simulink model "miniproject1901156"  (R2017b)
settings: Solver=VariableStepAuto  StartTime=0.0  StopTime=0.2  MaxStep=1e-4  RelTol=1e-3
undefined symbols (not defined in the file): D1, Delta
libraries: powerlib x32, powerlib_meascontrol x3
settings Model: Creator=DVCBD  LastModifiedBy=DVCBD

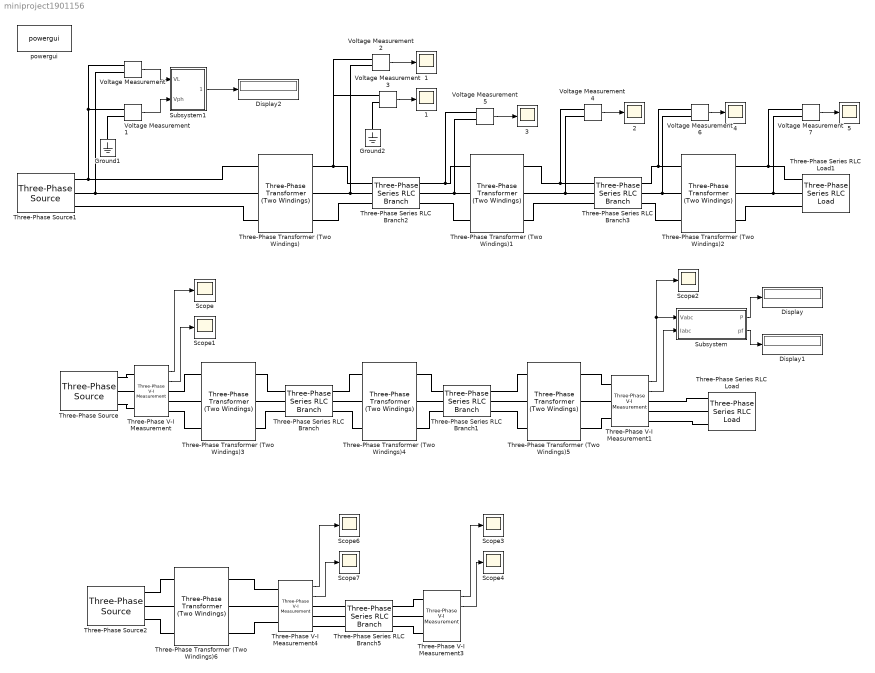
== system miniproject1901156 ==
   {1,1..5} (6 alike) : Scope
  Display : Display
  Display1 : Display
  Display2 : Display
  Ground1 : powerlib/Elements/Ground  LConnTagsString=a
  Ground2 : powerlib/Elements/Ground  LConnTagsString=a
  Scope{,1..4,6..7} (7 alike) : Scope
  Subsystem : Subsystem
  Subsystem1 : Subsystem
  Three-Phase Series RLC Branch{,1..3,5} (5 alike) : powerlib/Elements/Three-Phase Series RLC Branch  LConnTagsString=A|B|C  RConnTagsString=A|B|C  BranchType=RL  Resistance=(100+156)*0.01  Inductance=(100+156)*0.01  Capacitance=1e-6  Measurements=None
  Three-Phase Series RLC Load : powerlib/Elements/Three-Phase Series RLC Load  LConnTagsString=A|B|C  Configuration=Y (grounded)  NominalVoltage=1000  Vabc=[1e3 1e3 1e3]  Vabcp=[1e3 1e3 1e3]  NominalFrequency=50  UnbalancedPower=off  ActivePower=1e3  InductivePower=0.5e6  CapacitivePower=0  Pabc=[10e3 9e3 11e3]  QLabc=[100 90 110]  QCabc=[100 90 110]  Pabcp=[10e3 9e3 11e3]  QLabcp=[100 90 110]  QCabcp=[100 90 110]  Measurements=None  LoadType=constant Z
  Three-Phase Series RLC Load1 : powerlib/Elements/Three-Phase Series RLC Load  LConnTagsString=A|B|C  Configuration=Y (grounded)  NominalVoltage=1000  Vabc=[1e3 1e3 1e3]  Vabcp=[1e3 1e3 1e3]  NominalFrequency=50  UnbalancedPower=off  ActivePower=1e3  InductivePower=0.5e6  CapacitivePower=0  Pabc=[10e3 9e3 11e3]  QLabc=[100 90 110]  QCabc=[100 90 110]  Pabcp=[10e3 9e3 11e3]  QLabcp=[100 90 110]  QCabcp=[100 90 110]  Measurements=None  LoadType=constant Z
  Three-Phase Transformer (Two Windings) : powerlib/Elements/Three-Phase Transformer (Two Windings)  Winding1Connection=Delta (D1)  Winding2Connection=Yg  CoreType=Three single-phase transformers  SetSaturation=off  Hysteresis=off  DataFile='hysteresis'  SetInitialFlux=off  Measurements=None  UNITS=pu  NominalPower=[ 250e6 , 50 ]  Winding1=[ 11e3 , 0.002 , 0.08 ]  Winding2=[ 230e3 , 0.002 , 0.08 ]  Rm=500  Lm=500  L0=0.5  Saturation=[ 0,0 ; 0.0024,1.2 ; 1.0,1.52 ]  InitialFluxes=[ 0.8 , -0.8 , 0.7 ]  MoreParameters=off  BreakLoop=off  DataType=off  TransfoNumber=1
  Three-Phase Transformer (Two Windings)1 : powerlib/Elements/Three-Phase Transformer (Two Windings)  Winding1Connection=Yg  Winding2Connection=Delta (D1)  CoreType=Three single-phase transformers  SetSaturation=off  Hysteresis=off  DataFile='hysteresis'  SetInitialFlux=off  Measurements=None  UNITS=pu  NominalPower=[ 250e6 , 50 ]  Winding1=[ 230e3 , 0.002 , 0.08 ]  Winding2=[ 11e3 , 0.002 , 0.08 ]  Rm=500  Lm=500  L0=0.5  Saturation=[ 0,0 ; 0.0024,1.2 ; 1.0,1.52 ]  InitialFluxes=[ 0.8 , -0.8 , 0.7 ]  MoreParameters=off  BreakLoop=off  DataType=off  TransfoNumber=1
  Three-Phase Transformer (Two Windings)2 : powerlib/Elements/Three-Phase Transformer (Two Windings)  Winding1Connection=Yg  Winding2Connection=Yg  CoreType=Three single-phase transformers  SetSaturation=off  Hysteresis=off  DataFile='hysteresis'  SetInitialFlux=off  Measurements=None  UNITS=pu  NominalPower=[ 250e6 , 50 ]  Winding1=[ 11e3 , 0.002 , 0.08 ]  Winding2=[ 400 , 0.002 , 0.08 ]  Rm=500  Lm=500  L0=0.5  Saturation=[ 0,0 ; 0.0024,1.2 ; 1.0,1.52 ]  InitialFluxes=[ 0.8 , -0.8 , 0.7 ]  MoreParameters=off  BreakLoop=off  DataType=off  TransfoNumber=1
  Three-Phase Transformer (Two Windings)3 : powerlib/Elements/Three-Phase Transformer (Two Windings)  Winding1Connection=Delta (D1)  Winding2Connection=Yg  CoreType=Three single-phase transformers  SetSaturation=off  Hysteresis=off  DataFile='hysteresis'  SetInitialFlux=off  Measurements=None  UNITS=pu  NominalPower=[ 250e6 , 60 ]  Winding1=[ 11e3 , 0.002 , 0.08 ]  Winding2=[ 230e3 , 0.002 , 0.08 ]  Rm=500  Lm=500  L0=0.5  Saturation=[ 0,0 ; 0.0024,1.2 ; 1.0,1.52 ]  InitialFluxes=[ 0.8 , -0.8 , 0.7 ]  MoreParameters=off  BreakLoop=off  DataType=off  TransfoNumber=1
  Three-Phase Transformer (Two Windings)4 : powerlib/Elements/Three-Phase Transformer (Two Windings)  Winding1Connection=Yg  Winding2Connection=Delta (D1)  CoreType=Three single-phase transformers  SetSaturation=off  Hysteresis=off  DataFile='hysteresis'  SetInitialFlux=off  Measurements=None  UNITS=pu  NominalPower=[ 250e6 , 60 ]  Winding1=[ 230e3 , 0.002 , 0.08 ]  Winding2=[ 11e3 , 0.002 , 0.08 ]  Rm=500  Lm=500  L0=0.5  Saturation=[ 0,0 ; 0.0024,1.2 ; 1.0,1.52 ]  InitialFluxes=[ 0.8 , -0.8 , 0.7 ]  MoreParameters=off  BreakLoop=off  DataType=off  TransfoNumber=1
  Three-Phase Transformer (Two Windings)5 : powerlib/Elements/Three-Phase Transformer (Two Windings)  Winding1Connection=Yg  Winding2Connection=Yg  CoreType=Three single-phase transformers  SetSaturation=off  Hysteresis=off  DataFile='hysteresis'  SetInitialFlux=off  Measurements=None  UNITS=pu  NominalPower=[ 250e6 , 60 ]  Winding1=[ 11e3 , 0.002 , 0.08 ]  Winding2=[ 400 , 0.002 , 0.08 ]  Rm=500  Lm=500  L0=0.5  Saturation=[ 0,0 ; 0.0024,1.2 ; 1.0,1.52 ]  InitialFluxes=[ 0.8 , -0.8 , 0.7 ]  MoreParameters=off  BreakLoop=off  DataType=off  TransfoNumber=1
  Three-Phase Transformer (Two Windings)6 : powerlib/Elements/Three-Phase Transformer (Two Windings)  Winding1Connection=Delta (D1)  Winding2Connection=Yg  CoreType=Three single-phase transformers  SetSaturation=off  Hysteresis=off  DataFile='hysteresis'  SetInitialFlux=off  Measurements=None  UNITS=pu  NominalPower=[ 250e6 , 60 ]  Winding1=[ 11e3 , 0.002 , 0.08 ]  Winding2=[ 230e3 , 0.002 , 0.08 ]  Rm=500  Lm=500  L0=0.5  Saturation=[ 0,0 ; 0.0024,1.2 ; 1.0,1.52 ]  InitialFluxes=[ 0.8 , -0.8 , 0.7 ]  MoreParameters=off  BreakLoop=off  DataType=off  TransfoNumber=1
  Three-Phase V-I Measurement : powerlib/Measurements/Three-Phase V-I Measurement  VoltageMeasurement=phase-to-ground  SetLabelV=off  LabelV=Vabc  Vpu=off  VpuLL=off  CurrentMeasurement=yes  SetLabelI=off  LabelI=Iabc  Ipu=off  Pbase=100e6  Vbase=500e3  OutputType=Complex  PhasorSimulation=off  PSBequivalent=0
  Three-Phase V-I Measurement1 : powerlib/Measurements/Three-Phase V-I Measurement  VoltageMeasurement=phase-to-phase  SetLabelV=off  LabelV=Vabc  Vpu=off  VpuLL=off  CurrentMeasurement=yes  SetLabelI=off  LabelI=Iabc  Ipu=off  Pbase=100e6  Vbase=500e3  OutputType=Complex  PhasorSimulation=off  PSBequivalent=0
  Three-Phase V-I Measurement3 : powerlib/Measurements/Three-Phase V-I Measurement  VoltageMeasurement=phase-to-phase  SetLabelV=off  LabelV=Vabc  Vpu=off  VpuLL=off  CurrentMeasurement=yes  SetLabelI=off  LabelI=Iabc  Ipu=off  Pbase=100e6  Vbase=500e3  OutputType=Complex  PhasorSimulation=off  PSBequivalent=0
  Three-Phase V-I Measurement4 : powerlib/Measurements/Three-Phase V-I Measurement  VoltageMeasurement=phase-to-ground  SetLabelV=off  LabelV=Vabc  Vpu=off  VpuLL=off  CurrentMeasurement=yes  SetLabelI=off  LabelI=Iabc  Ipu=off  Pbase=100e6  Vbase=500e3  OutputType=Complex  PhasorSimulation=off  PSBequivalent=0
  Three-Phase Source : powerlib/Electrical Sources/Three-Phase Source  InternalConnection=Yg  VoltagePhases=off  Voltage=11000  PhaseAngle=0  Voltage_phases=[25e3 25e3 25e3]/sqrt(3)  PhaseAngles_phases=[0 -120 +120]  Frequency=50  NonIdealSource=on  SpecifyImpedance=off  Resistance=0  Inductance=0  ShortCircuitLevel=100e6  BaseVoltage=25e3  XRratio=7  BusType=swing  Pref=10e3  Qref=0  Prefabc=[10e3, 10e3, 10e3]  Qrefabc=[0, 0, 0]  Qmin=-inf  Qmax=inf
  Three-Phase Source1 : powerlib/Electrical Sources/Three-Phase Source  InternalConnection=Yg  VoltagePhases=off  Voltage=11000  PhaseAngle=0  Voltage_phases=[25e3 25e3 25e3]/sqrt(3)  PhaseAngles_phases=[0 -120 +120]  Frequency=50  NonIdealSource=on  SpecifyImpedance=off  Resistance=0  Inductance=0  ShortCircuitLevel=100e6  BaseVoltage=25e3  XRratio=7  BusType=swing  Pref=10e3  Qref=0  Prefabc=[10e3, 10e3, 10e3]  Qrefabc=[0, 0, 0]  Qmin=-inf  Qmax=inf
  Three-Phase Source2 : powerlib/Electrical Sources/Three-Phase Source  InternalConnection=Yg  VoltagePhases=off  Voltage=11000  PhaseAngle=0  Voltage_phases=[25e3 25e3 25e3]/sqrt(3)  PhaseAngles_phases=[0 -120 +120]  Frequency=50  NonIdealSource=on  SpecifyImpedance=off  Resistance=0  Inductance=0  ShortCircuitLevel=100e6  BaseVoltage=25e3  XRratio=7  BusType=swing  Pref=10e3  Qref=0  Prefabc=[10e3, 10e3, 10e3]  Qrefabc=[0, 0, 0]  Qmin=-inf  Qmax=inf
  Voltage Measurement{,1..7} (8 alike) : powerlib/Measurements/Voltage Measurement  PhasorSimulation=off  OutputType=Complex  PSBequivalent=0
  powergui : powerlib/powergui  Priority=1  SimulationMode=Continuous  SampleTime=50e-6  frequency=60  Iterations=50  frequencyindice=50  Pbase=100e6  ErrMax=1e-4  UnitsV=kV  UnitsW=MW  buscounter=0  FunctionMessages=off  echomessages=off  EnableUseOfTLC=off  CurrentSourceSwitches=off  DisableSnubberDevices=off  DisableRonSwitches=off  DisableVfSwitches=off  DisplayEquations=off  SolverType=Tustin/Backward Euler (TBE)  Interpol=off  ExternalGateDelay=off  methode=off  Ts=100  x0status=blocks  SPID=on  SwTol=0  HookPort=off  RestoreLinks=warning  ResistiveCurrentMeasurement=off  Frange=[0:2:500]  Ylog=off  Xlog=on  ShowGrid=off  save=off  variable=ZData  structure=0  ZoomFFT=off  StartTime=0.0  cycles=1  DisplayStyle=1  fundamental=60  FreqAxis=off  MaxFrequency=1000  frequencyindicesteady=1  RmsSteady=1  display=off
  wires:
  Three-Phase V-I Measurement/1 -> Scope/1
  Three-Phase V-I Measurement/2 -> Scope1/1
  Three-Phase V-I Measurement1/2 -> Subsystem/2(Iabc)
  Three-Phase V-I Measurement1/1 -> Scope2/1, Subsystem/1(Vabc)
  Subsystem/1(P) -> Display/1
  Subsystem/2(pf) -> Display1/1
  Voltage Measurement3/1 -> " 1"/1
  Voltage Measurement2/1 -> " 1"/1
  Voltage Measurement4/1 -> " 2"/1
  Voltage Measurement5/1 -> " 3"/1
  Voltage Measurement6/1 -> " 4"/1
  Voltage Measurement7/1 -> " 5"/1
  Voltage Measurement/1 -> Subsystem1/1(VL)
  Voltage Measurement1/1 -> Subsystem1/2(Vph)
  Subsystem1/1(VL/Vph) -> Display2/1
  Three-Phase V-I Measurement4/2 -> Scope7/1
  Three-Phase V-I Measurement4/1 -> Scope6/1
  Three-Phase V-I Measurement3/1 -> Scope3/1
  Three-Phase V-I Measurement3/2 -> Scope4/1
  connections:
  Three-Phase Source/RConn1 -- Three-Phase V-I Measurement/LConn1
  Three-Phase Source/RConn2 -- Three-Phase V-I Measurement/LConn2
  Three-Phase Source/RConn3 -- Three-Phase V-I Measurement/LConn3
  Three-Phase Transformer (Two Windings)3/LConn1 -- Three-Phase V-I Measurement/RConn1
  Three-Phase Transformer (Two Windings)3/LConn2 -- Three-Phase V-I Measurement/RConn2
  Three-Phase Transformer (Two Windings)3/LConn3 -- Three-Phase V-I Measurement/RConn3
  Three-Phase Series RLC Branch/LConn2 -- Three-Phase Transformer (Two Windings)3/RConn2
  Three-Phase Series RLC Branch/LConn1 -- Three-Phase Transformer (Two Windings)3/RConn1
  Three-Phase Series RLC Branch/LConn3 -- Three-Phase Transformer (Two Windings)3/RConn3
  Three-Phase Series RLC Branch/RConn2 -- Three-Phase Transformer (Two Windings)4/LConn2
  Three-Phase Series RLC Branch/RConn1 -- Three-Phase Transformer (Two Windings)4/LConn1
  Three-Phase Series RLC Branch/RConn3 -- Three-Phase Transformer (Two Windings)4/LConn3
  Three-Phase Transformer (Two Windings)4/RConn2 -- Three-Phase Series RLC Branch1/LConn2
  Three-Phase Transformer (Two Windings)4/RConn1 -- Three-Phase Series RLC Branch1/LConn1
  Three-Phase Transformer (Two Windings)4/RConn3 -- Three-Phase Series RLC Branch1/LConn3
  Three-Phase Series RLC Branch1/RConn2 -- Three-Phase Transformer (Two Windings)5/LConn2
  Three-Phase Series RLC Branch1/RConn1 -- Three-Phase Transformer (Two Windings)5/LConn1
  Three-Phase Series RLC Branch1/RConn3 -- Three-Phase Transformer (Two Windings)5/LConn3
  Three-Phase Transformer (Two Windings)5/RConn2 -- Three-Phase V-I Measurement1/LConn2
  Three-Phase Transformer (Two Windings)5/RConn1 -- Three-Phase V-I Measurement1/LConn1
  Three-Phase Transformer (Two Windings)5/RConn3 -- Three-Phase V-I Measurement1/LConn3
  Three-Phase Series RLC Load/LConn2 -- Three-Phase V-I Measurement1/RConn2
  Three-Phase V-I Measurement1/RConn1 -- Three-Phase Series RLC Load/LConn1
  Three-Phase V-I Measurement1/RConn3 -- Three-Phase Series RLC Load/LConn3
  Three-Phase Source1/RConn2 -- Three-Phase Transformer (Two Windings)/LConn2 -- Voltage Measurement/LConn2
  Three-Phase Transformer (Two Windings)/LConn3 -- Three-Phase Source1/RConn3
  Ground2/LConn1 -- Voltage Measurement3/LConn2
  Three-Phase Series RLC Branch2/LConn1 -- Voltage Measurement3/LConn1 -- Voltage Measurement2/LConn1 -- Three-Phase Transformer (Two Windings)/RConn1
  Three-Phase Series RLC Branch2/LConn2 -- Three-Phase Transformer (Two Windings)/RConn2 -- Voltage Measurement2/LConn2
  Three-Phase Transformer (Two Windings)/RConn3 -- Three-Phase Series RLC Branch2/LConn3
  Three-Phase Series RLC Branch2/RConn1 -- Three-Phase Transformer (Two Windings)1/LConn1 -- Voltage Measurement5/LConn1
  Three-Phase Series RLC Branch2/RConn2 -- Three-Phase Transformer (Two Windings)1/LConn2 -- Voltage Measurement5/LConn2
  Three-Phase Transformer (Two Windings)1/LConn3 -- Three-Phase Series RLC Branch2/RConn3
  Three-Phase Series RLC Branch3/LConn2 -- Three-Phase Transformer (Two Windings)1/RConn2 -- Voltage Measurement4/LConn2
  Three-Phase Series RLC Branch3/LConn1 -- Three-Phase Transformer (Two Windings)1/RConn1 -- Voltage Measurement4/LConn1
  Three-Phase Series RLC Branch3/LConn3 -- Three-Phase Transformer (Two Windings)1/RConn3
  Three-Phase Series RLC Branch3/RConn2 -- Three-Phase Transformer (Two Windings)2/LConn2 -- Voltage Measurement6/LConn2
  Three-Phase Series RLC Branch3/RConn1 -- Three-Phase Transformer (Two Windings)2/LConn1 -- Voltage Measurement6/LConn1
  Three-Phase Transformer (Two Windings)2/LConn3 -- Three-Phase Series RLC Branch3/RConn3
  Three-Phase Series RLC Load1/LConn2 -- Voltage Measurement7/LConn2 -- Three-Phase Transformer (Two Windings)2/RConn2
  Voltage Measurement7/LConn1 -- Three-Phase Series RLC Load1/LConn1 -- Three-Phase Transformer (Two Windings)2/RConn1
  Three-Phase Series RLC Load1/LConn3 -- Three-Phase Transformer (Two Windings)2/RConn3
  Voltage Measurement/LConn1 -- Voltage Measurement1/LConn1 -- Three-Phase Transformer (Two Windings)/LConn1 -- Three-Phase Source1/RConn1
  Ground1/LConn1 -- Voltage Measurement1/LConn2
  Three-Phase V-I Measurement3/LConn3 -- Three-Phase Series RLC Branch5/RConn3
  Three-Phase V-I Measurement3/LConn1 -- Three-Phase Series RLC Branch5/RConn1
  Three-Phase V-I Measurement3/LConn2 -- Three-Phase Series RLC Branch5/RConn2
  Three-Phase Source2/RConn2 -- Three-Phase Transformer (Two Windings)6/LConn2
  Three-Phase Source2/RConn1 -- Three-Phase Transformer (Two Windings)6/LConn1
  Three-Phase Source2/RConn3 -- Three-Phase Transformer (Two Windings)6/LConn3
  Three-Phase Transformer (Two Windings)6/RConn2 -- Three-Phase V-I Measurement4/LConn2
  Three-Phase Transformer (Two Windings)6/RConn1 -- Three-Phase V-I Measurement4/LConn1
  Three-Phase Transformer (Two Windings)6/RConn3 -- Three-Phase V-I Measurement4/LConn3
  Three-Phase Series RLC Branch5/LConn1 -- Three-Phase V-I Measurement4/RConn1
  Three-Phase Series RLC Branch5/LConn2 -- Three-Phase V-I Measurement4/RConn2
  Three-Phase Series RLC Branch5/LConn3 -- Three-Phase V-I Measurement4/RConn3

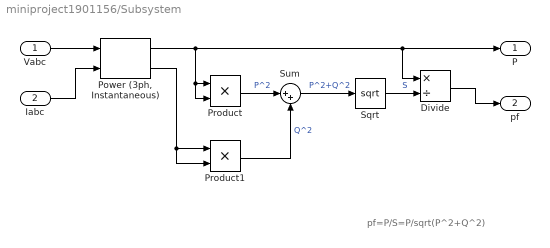
== system miniproject1901156/Subsystem ==
  note: pf=P/S=P/sqrt(P^2+Q^2)
  Vabc : Inport
  Iabc : Inport  Port=2
  Divide : Product  Inputs=*/
  "Power (3ph, Instantaneous)" : powerlib_meascontrol/Measurements/Power (3ph, Instantaneous)
      settings: SourceProductName=Simscape Power Systems
  Product : Product
  Product1 : Product
  Sqrt : Sqrt  SaturateOnIntegerOverflow=on
  Sum : Sum  Inputs=|++
  P : Outport
  pf : Outport  Port=2
  wires:
  Vabc/1 -> "Power (3ph, Instantaneous)"/1
  Iabc/1 -> "Power (3ph, Instantaneous)"/2
  "Power (3ph, Instantaneous)"/1 -> Product/2, Product/1, Divide/1, P/1
  Divide/1 -> pf/1
  Sqrt/1 -> Divide/2  "S"
  Sum/1 -> Sqrt/1  "P^2+Q^2"
  Product/1 -> Sum/1  "P^2"
  Product1/1 -> Sum/2  "Q^2"
  "Power (3ph, Instantaneous)"/2 -> Product1/2, Product1/1

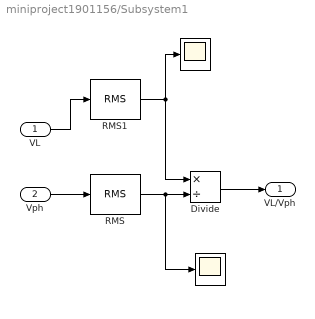
== system miniproject1901156/Subsystem1 ==
  VL : Inport
  Vph : Inport  Port=2
  " " : Scope
  " " : Scope
  Divide : Product  Inputs=*/
  RMS : powerlib_meascontrol/Measurements/RMS  TrueRMS=on  Freq=50  RMSInit=120  Ts=0
  RMS1 : powerlib_meascontrol/Measurements/RMS  TrueRMS=on  Freq=50  RMSInit=120  Ts=0
  VL/Vph : Outport
  wires:
  RMS1/1 -> Divide/1, " "/1
  Divide/1 -> VL/Vph/1
  RMS/1 -> Divide/2, " "/1
  Vph/1 -> RMS/1
  VL/1 -> RMS1/1
